simulink library "ayazPlant_cl"  (R2018b)
settings: Solver=VariableStepAuto  StartTime=0.0  StopTime=10.0  RelTol=1e-3
undefined symbols (not defined in the file or in its folder): sim_param
libraries: threeTethers_cl x1, ayazLiftingBody_cl x1, ayazWinches_cl x1, threeTetherGroundStation_cl x1
settings Model: Creator=mcobb  LastModifiedBy=mcobb

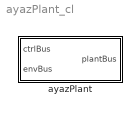
== system ayazPlant_cl ==
  ayazPlant : Subsystem

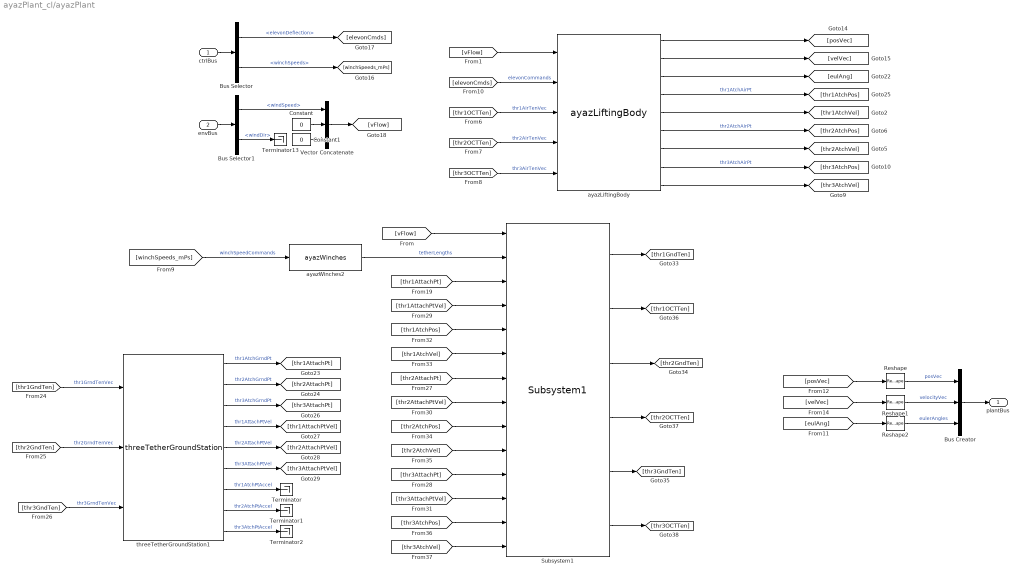
== system ayazPlant_cl/ayazPlant ==
  ctrlBus : Inport  OutDataTypeStr=Bus: ctrlBus
  envBus : Inport  Port=2  OutDataTypeStr=Bus: envBus
  Bus Creator : BusCreator  Inputs=3  OutDataTypeStr=Bus: plantBus
  Bus Selector : BusSelector  OutputSignals=elevonDeflection,winchSpeeds
  Bus Selector1 : BusSelector  OutputSignals=windSpeed,windDir
  Constant : Constant  Value=0
  Constant1 : Constant  Value=0
  Reshape : Reshape  OutputDimensionality=Column vector (2-D)
  Reshape1 : Reshape  OutputDimensionality=Column vector (2-D)
  Reshape2 : Reshape  OutputDimensionality=Column vector (2-D)
  Subsystem1 : threeTethers_cl/Subsystem1  SystemSampleTime=-1
  Terminator{,1..2,13} (4 alike) : Terminator
  Vector Concatenate : Concatenate  NumInputs=3
  ayazLiftingBody : ayazLiftingBody_cl/ayazLiftingBody  SystemSampleTime=-1
  ayazWinches2 : ayazWinches_cl/ayazWinches  maxSpeed=maxWinchSpeed  maxAccel=maxWinchAccel  timeConst=1  tetherLengths=unstretched_l
  threeTetherGroundStation1 : threeTetherGroundStation_cl/threeTetherGroundStation  fixed=1  J=sim_param.platform_param.platform_Izz  b=sim_param.platform_param.platform_damping  posVec=[0 0 0]  thr1AttachPt=sim_param.tether_imp_nodes.R11_g  thr2AttachPt=sim_param.tether_imp_nodes.R21_g  thr3AttachPt=sim_param.tether_imp_nodes.R31_g  initAngPos=ini_platform_ang  initAngVel=ini_platform_vel
  plantBus : Outport  OutDataTypeStr=Bus: plantBus
  wires:
  ayazLiftingBody/1 -> [posVec]
  ayazLiftingBody/2 -> [velVec]
  [vFlow] -> ayazLiftingBody/1
  [thr1OCTTen] -> ayazLiftingBody/3  "thr1AirTenVec"
  [thr2OCTTen] -> ayazLiftingBody/4  "thr2AirTenVec"
  [thr3OCTTen] -> ayazLiftingBody/5  "thr3AirTenVec"
  [elevonCmds] -> ayazLiftingBody/2  "elevonCommands"
  envBus/1 -> Bus Selector1/1
  ctrlBus/1 -> Bus Selector/1
  Bus Selector1/2 -> Terminator13/1  "<windDir>"
  Bus Selector/1 -> [elevonCmds]  "<elevonDeflection>"
  Bus Selector1/1 -> Vector Concatenate/1  "<windSpeed>"
  Bus Selector/2 -> [winchSpeeds_mPs]  "<winchSpeeds>"
  Bus Creator/1 -> plantBus/1
  Reshape/1 -> Bus Creator/1  "posVec"
  Reshape2/1 -> Bus Creator/3  "eulerAngles"
  Reshape1/1 -> Bus Creator/2  "velocityVec"
  Vector Concatenate/1 -> [vFlow]
  Constant/1 -> Vector Concatenate/2
  Constant1/1 -> Vector Concatenate/3
  ayazLiftingBody/3 -> [eulAng]
  ayazLiftingBody/4 -> [thr1AtchPos]  "thr1AtchAirPt"
  ayazLiftingBody/5 -> [thr1AtchVel]
  ayazLiftingBody/6 -> [thr2AtchPos]  "thr2AtchAirPt"
  ayazLiftingBody/7 -> [thr2AtchVel]
  ayazLiftingBody/8 -> [thr3AtchPos]  "thr3AtchAirPt"
  ayazLiftingBody/9 -> [thr3AtchVel]
  threeTetherGroundStation1/9 -> Terminator2/1  "thr3AtchPtAccel"
  threeTetherGroundStation1/6 -> [thr3AttachPtVel]  "thr3AttachPtVel"
  threeTetherGroundStation1/5 -> [thr2AttachPtVel]  "thr2AttachPtVel"
  threeTetherGroundStation1/8 -> Terminator1/1  "thr2AtchPtAccel"
  threeTetherGroundStation1/4 -> [thr1AttachPtVel]  "thr1AttachPtVel"
  threeTetherGroundStation1/2 -> [thr2AttachPt]  "thr2AtchGrndPt"
  threeTetherGroundStation1/3 -> [thr3AttachPt]  "thr3AtchGrndPt"
  threeTetherGroundStation1/1 -> [thr1AttachPt]  "thr1AtchGrndPt"
  ayazWinches2/1 -> Subsystem1/2  "tetherLengths"
  [thr2GndTen] -> threeTetherGroundStation1/2  "thr2GrndTenVec"
  [winchSpeeds_mPs] -> ayazWinches2/1  "winchSpeedCommands"
  [thr3GndTen] -> threeTetherGroundStation1/3  "thr3GrndTenVec"
  [thr1GndTen] -> threeTetherGroundStation1/1  "thr1GrndTenVec"
  threeTetherGroundStation1/7 -> Terminator/1  "thr1AtchPtAccel"
  [vFlow] -> Subsystem1/1
  [thr1AttachPt] -> Subsystem1/3
  [thr2AttachPt] -> Subsystem1/7
  [thr3AttachPt] -> Subsystem1/11
  [thr3AttachPtVel] -> Subsystem1/12
  [thr2AttachPtVel] -> Subsystem1/8
  [thr1AttachPtVel] -> Subsystem1/4
  [thr1AtchPos] -> Subsystem1/5
  [thr3AtchVel] -> Subsystem1/14
  [thr3AtchPos] -> Subsystem1/13
  [thr2AtchVel] -> Subsystem1/10
  [thr2AtchPos] -> Subsystem1/9
  [thr1AtchVel] -> Subsystem1/6
  Subsystem1/1 -> [thr1GndTen]
  Subsystem1/2 -> [thr1OCTTen]
  Subsystem1/3 -> [thr2GndTen]
  Subsystem1/4 -> [thr2OCTTen]
  Subsystem1/6 -> [thr3OCTTen]
  Subsystem1/5 -> [thr3GndTen]
  [posVec] -> Reshape/1
  [velVec] -> Reshape1/1
  [eulAng] -> Reshape2/1
